simulink model "LineGotoFromDemo"  (Simulink 7.8)
settings: Solver=ode45  StartTime=0.0  StopTime=10.0  RelTol=1e-3
settings Model: Creator=T6684MB  LastModifiedBy=T6684MB

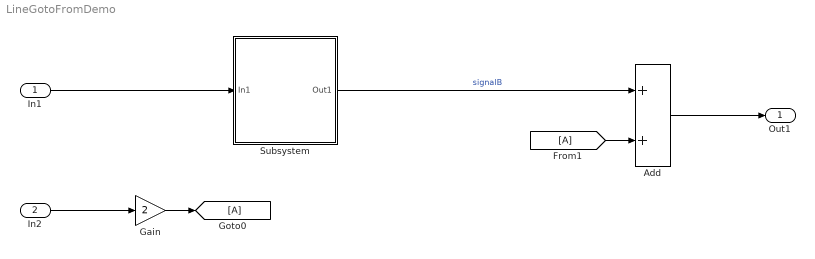
== system LineGotoFromDemo ==
  In1 : Inport
  In2 : Inport  Port=2
  Add : Sum
  Gain : Gain  Gain=2
  Subsystem : Subsystem
  Out1 : Outport
  wires:
  Add/1 -> Out1/1
  In2/1 -> Gain/1
  In1/1 -> Subsystem/1(In1)
  Subsystem/1(Out1) -> Add/1  "signalB"
  Gain/1 -> [A]
  [A] -> Add/2

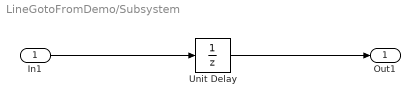
== system LineGotoFromDemo/Subsystem ==
  In1 : Inport
  Unit Delay : UnitDelay  SampleTime=-1
  Out1 : Outport
  wires:
  In1/1 -> Unit Delay/1
  Unit Delay/1 -> Out1/1
